simulink model "VehCtrl20260630_18B"  (R2018b)
settings: Solver=FixedStepAuto  StartTime=0.0  StopTime=inf  FixedStep=0.005  RelTol=1e-3
InitFcn:
  | mbd_mpc_consistency_checks(bdroot(gcs));
undefined symbols (not defined in the file): ANG_DEAD, BMS_NormalPwr, BrakeDeadZone, BrkPrsByBrkPct_TB_X, BrkPrsByBrkPct_TB_Y, DELAY_DISCHARGE, DELAY_RCUOFF, DRV_BACKWARD, DRV_BRAKE, DRV_FORWARD, DRV_NEUTRAL, DRV_PARK, DRV_UNPARK, DRV_ZEROTURN, EPB_LOCK, EPB_UNLOCK, ExtraLoadPwr, FanOff, fifo_0_vect, fifo_1_vect, HiFanReq, HV_finished, HV_No_Active, HV_POWER_OFF, HV_POWER_ON, HVDown, HVON, KaTLS_v_DrgUp_X_VehSpd, KeFTM_s_Way1OffDlyTime, KeFTM_TK_Way1CoolLv2OffBatTemp, KeFTM_TK_Way1CoolLv2OffMtrTemp, KeFTM_TK_Way1CoolLv2OnBatTemp, KeFTM_TK_Way1CoolLv2OnMtrTemp, KeFTM_TK_Way1CoolLv3OffBatTemp, KeFTM_TK_Way1CoolLv3OffMtrTemp, KeFTM_TK_Way1CoolLv3OnBatTemp, KeFTM_TK_Way1CoolLv3OnMtrTemp, KeFTM_TK_Way1CoolLv4OffBatTemp, KeFTM_TK_Way1CoolLv4OffMtrTemp, KeFTM_TK_Way1CoolLv4OnBatTemp, KeFTM_TK_Way1CoolLv4OnMtrTemp, Kp1, Kp2, LowFanReq, LQFP, MtrCmdGainFL, MtrCmdGainFR, MtrCmdGainRL, MtrCmdGainRR, MtrPwrFactor_RCU, MtrPwrHighToMidThd, MtrPwrLowToMidThd, MtrPwrMidToHighThd, MtrPwrMidToLowThd, MtrTrqMax, PCT_DEAD, Precharge, PTO_1000, PTO_540, pts1_fifo_0_vect ... (+32)
libraries: mbd_mpc574x_ec_toolbox x175, simulink x110, canmsglib x70
(part 9 of 15)

== system VehCtrl20260630_18B/SigIn/CAN1/BMS_CellVoltageCycTx/UNPACK ==
  ID : Inport
  data : Inport  Port=2
  length : Inport  Port=3
  timestamp : Inport  Port=4
  Action Port : ActionPort  ActionType=case
  Bus Creator : BusCreator  Inputs=7  OutDataTypeStr=Bus: CAN_MESSAGE_BUS  NonVirtualBus=on
  Bus Creator1 : BusCreator  Inputs=5
  CAN Unpack6 : canmsglib/CAN Unpack  CANdbFile=D:\VCU\VCU_AgriculturalMachinery_ChangChun\CAN协议8.4\BMS\BMS_DBC_Sheet1.dbc  MsgList=BMS_CellVoltageCycTx  MsgName=BMS_CellVoltageCycTx  MsgIDType=Extended (29-bit identifier)  MsgIdentifier=404760903  MsgLength=8  SignalInfo=BMS_CellVolGroupNum$12$12$2$2$1$0$1$0$1$4095$#BMS_CellVol_n0$16$12$2$2$1$0$2.000000e-03$0$0$5$#BMS_CellVol_n1$36$12$2$2$1$0$2.000000e-03$0$0$5$#BMS_CellVol_n2$40$12$2$2$1$0$2.000000e-03$0$0$5$#BMS_CellVol_n3$60$12$2$2$1$0$2.000000e-03$0$0$5$#  NSignals=5  IDPort=off  TimestampPort=off  ErrorPort=off  RemotePort=off  LengthPort=off  StatusPort=off  StartBits=str2num('[int32(12);int32(16);int32(36);int32(40);int32(60)]')  SignalSizes=str2num('[int32(12);int32(12);int32(12);int32(12);int32(12)]')  ByteOrders=str2num('[int32(2);int32(2);int32(2);int32(2);int32(2)]')  DataTypes=str2num('[int32(2);int32(2);int32(2);int32(2);int32(2)]')  MultiplexTypes=str2num('[int32(1);int32(1);int32(1);int32(1);int32(1)]')  MultiplexValues=str2num('[double(0);double(0);double(0);double(0);double(0)]')  Factors=str2num('[double(1);double(2.000000e-03);double(2.000000e-03);double(2.000000e-03);double(2.000000e-03)]')  Offsets=str2num('[double(0);double(0);double(0);double(0);double(0)]')  Minimums=str2num('[double(1);double(0);double(0);double(0);double(0)]')  Maximums=str2num('[double(4095);double(5);double(5);double(5);double(5)]')  ApplyMinMax=off
      settings: SourceProductName=Simulink Real-Time  SourceProductBaseCode=XP  DataFormat=CANdb specified signals
  Constant1 : Constant  OutDataTypeStr=uint8
  Constant4 : Constant  Value=0  OutDataTypeStr=uint8
  Constant5 : Constant  Value=0  OutDataTypeStr=uint8
  Data Type Conversion{,14..15,17} (4 alike) : DataTypeConversion  OutDataTypeStr=uint8
  Data Type Conversion{1..4,60} (5 alike) : DataTypeConversion  OutDataTypeStr=single
  Data Type Conversion18 : DataTypeConversion  OutDataTypeStr=uint32
  Data Type Conversion19 : DataTypeConversion  OutDataTypeStr=double
  Message : Outport
  wires:
  Data Type Conversion15/1 -> Bus Creator/3  "Remote"
  Data Type Conversion14/1 -> Bus Creator/2  "Length"
  Data Type Conversion/1 -> Bus Creator/1  "Extended"
  Bus Creator/1 -> CAN Unpack6/1  "CAN_Msg_In"
  Data Type Conversion17/1 -> Bus Creator/4  "Error"
  timestamp/1 -> Data Type Conversion19/1
  Data Type Conversion19/1 -> Bus Creator/6  "Timestamp"
  ID/1 -> Data Type Conversion18/1
  Constant5/1 -> Data Type Conversion17/1
  Constant1/1 -> Data Type Conversion/1
  Data Type Conversion18/1 -> Bus Creator/5  "ID"
  data/1 -> Bus Creator/7  "Data"
  length/1 -> Data Type Conversion14/1
  Constant4/1 -> Data Type Conversion15/1
  CAN Unpack6/1 -> Data Type Conversion1/1
  CAN Unpack6/2 -> Data Type Conversion60/1
  CAN Unpack6/3 -> Data Type Conversion4/1
  CAN Unpack6/4 -> Data Type Conversion3/1
  CAN Unpack6/5 -> Data Type Conversion2/1
  Data Type Conversion1/1 -> Bus Creator1/1  "BMS_CellVolGroupNum"
  Data Type Conversion60/1 -> Bus Creator1/2  "BMS_CellVol_n0"
  Data Type Conversion4/1 -> Bus Creator1/3  "BMS_CellVol_n1"
  Data Type Conversion3/1 -> Bus Creator1/4  "BMS_CellVol_n2"
  Data Type Conversion2/1 -> Bus Creator1/5  "BMS_CellVol_n3"
  Bus Creator1/1 -> Message/1

== system VehCtrl20260630_18B/SigIn/CAN1/BMS_ExtremeCellVoltage/UNPACK ==
  ID : Inport
  data : Inport  Port=2
  length : Inport  Port=3
  timestamp : Inport  Port=4
  Action Port : ActionPort  ActionType=case
  Bus Creator : BusCreator  Inputs=7  OutDataTypeStr=Bus: CAN_MESSAGE_BUS  NonVirtualBus=on
  Bus Creator1 : BusCreator  Inputs=4
  CAN Unpack6 : canmsglib/CAN Unpack  CANdbFile=D:\VCU\VCU_AgriculturalMachinery_ChangChun\CAN协议8.4\BMS\BMS_DBC_Sheet1.dbc  MsgList=BMS_ExtremeCellVoltage  MsgName=BMS_ExtremeCellVoltage  MsgIDType=Extended (29-bit identifier)  MsgIdentifier=402794823  MsgLength=8  SignalInfo=BMS_MaxCellVoltage$16$12$2$2$1$0$2.000000e-03$0$0$5$#BMS_MaxCellVoltageNum$34$10$2$2$1$0$1$0$0$1023$#BMS_MinCellVoltage$54$12$2$2$1$0$2.000000e-03$0$0$5$#BMS_MinCellVoltageNum$56$10$2$2$1$0$1$0$0$1023$#  NSignals=4  IDPort=off  TimestampPort=off  ErrorPort=off  RemotePort=off  LengthPort=off  StatusPort=off  StartBits=str2num('[int32(16);int32(34);int32(54);int32(56)]')  SignalSizes=str2num('[int32(12);int32(10);int32(12);int32(10)]')  ByteOrders=str2num('[int32(2);int32(2);int32(2);int32(2)]')  DataTypes=str2num('[int32(2);int32(2);int32(2);int32(2)]')  MultiplexTypes=str2num('[int32(1);int32(1);int32(1);int32(1)]')  MultiplexValues=str2num('[double(0);double(0);double(0);double(0)]')  Factors=str2num('[double(2.000000e-03);double(1);double(2.000000e-03);double(1)]')  Offsets=str2num('[double(0);double(0);double(0);double(0)]')  Minimums=str2num('[double(0);double(0);double(0);double(0)]')  Maximums=str2num('[double(5);double(1023);double(5);double(1023)]')  ApplyMinMax=off
      settings: SourceProductName=Simulink Real-Time  SourceProductBaseCode=XP  DataFormat=CANdb specified signals
  Constant1 : Constant  OutDataTypeStr=uint8
  Constant4 : Constant  Value=0  OutDataTypeStr=uint8
  Constant5 : Constant  Value=0  OutDataTypeStr=uint8
  Data Type Conversion{,14..15,17} (4 alike) : DataTypeConversion  OutDataTypeStr=uint8
  Data Type Conversion{1..3,60} (4 alike) : DataTypeConversion  OutDataTypeStr=single
  Data Type Conversion18 : DataTypeConversion  OutDataTypeStr=uint32
  Data Type Conversion19 : DataTypeConversion  OutDataTypeStr=double
  Message : Outport
  wires:
  Bus Creator1/1 -> Message/1
  Data Type Conversion15/1 -> Bus Creator/3  "Remote"
  Data Type Conversion14/1 -> Bus Creator/2  "Length"
  Data Type Conversion/1 -> Bus Creator/1  "Extended"
  Bus Creator/1 -> CAN Unpack6/1  "CAN_Msg_In"
  Data Type Conversion17/1 -> Bus Creator/4  "Error"
  timestamp/1 -> Data Type Conversion19/1
  Data Type Conversion19/1 -> Bus Creator/6  "Timestamp"
  ID/1 -> Data Type Conversion18/1
  Constant5/1 -> Data Type Conversion17/1
  Constant1/1 -> Data Type Conversion/1
  Data Type Conversion18/1 -> Bus Creator/5  "ID"
  data/1 -> Bus Creator/7  "Data"
  length/1 -> Data Type Conversion14/1
  Constant4/1 -> Data Type Conversion15/1
  Data Type Conversion3/1 -> Bus Creator1/4  "BMS_MinCellVoltageNum"
  Data Type Conversion2/1 -> Bus Creator1/3  "BMS_MinCellVoltage"
  CAN Unpack6/1 -> Data Type Conversion1/1
  CAN Unpack6/2 -> Data Type Conversion60/1
  CAN Unpack6/4 -> Data Type Conversion3/1
  CAN Unpack6/3 -> Data Type Conversion2/1
  Data Type Conversion1/1 -> Bus Creator1/1  "BMS_MaxCellVoltage"
  Data Type Conversion60/1 -> Bus Creator1/2  "BMS_MaxCellVoltageNum"

== system VehCtrl20260630_18B/SigIn/CAN1/BMS_ExtremeTemp/UNPACK ==
  ID : Inport
  data : Inport  Port=2
  length : Inport  Port=3
  timestamp : Inport  Port=4
  Action Port : ActionPort  ActionType=case
  Bus Creator : BusCreator  Inputs=7  OutDataTypeStr=Bus: CAN_MESSAGE_BUS  NonVirtualBus=on
  Bus Creator1 : BusCreator  Inputs=4
  CAN Unpack6 : canmsglib/CAN Unpack  CANdbFile=D:\VCU\VCU_AgriculturalMachinery_ChangChun\CAN协议8.4\BMS\BMS_DBC_Sheet1.dbc  MsgList=BMS_ExtremeTemp  MsgName=BMS_ExtremeTemp  MsgIDType=Extended (29-bit identifier)  MsgIdentifier=402860359  MsgLength=8  SignalInfo=BMS_MaxBatteryTemp$8$8$2$2$1$0$1$-40$-40$125$#BMS_MaxBatteryTempNum$28$8$2$2$1$0$1$0$0$255$#BMS_MinBatteryTemp$36$8$2$2$1$0$1$-40$-40$125$#BMS_MinBatteryTempNum$40$8$2$2$1$0$1$0$0$255$#  NSignals=4  IDPort=off  TimestampPort=off  ErrorPort=off  RemotePort=off  LengthPort=off  StatusPort=off  StartBits=str2num('[int32(8);int32(28);int32(36);int32(40)]')  SignalSizes=str2num('[int32(8);int32(8);int32(8);int32(8)]')  ByteOrders=str2num('[int32(2);int32(2);int32(2);int32(2)]')  DataTypes=str2num('[int32(2);int32(2);int32(2);int32(2)]')  MultiplexTypes=str2num('[int32(1);int32(1);int32(1);int32(1)]')  MultiplexValues=str2num('[double(0);double(0);double(0);double(0)]')  Factors=str2num('[double(1);double(1);double(1);double(1)]')  Offsets=str2num('[double(-40);double(0);double(-40);double(0)]')  Minimums=str2num('[double(-40);double(0);double(-40);double(0)]')  Maximums=str2num('[double(125);double(255);double(125);double(255)]')  ApplyMinMax=off
      settings: SourceProductName=Simulink Real-Time  SourceProductBaseCode=XP  DataFormat=CANdb specified signals
  Constant1 : Constant  OutDataTypeStr=uint8
  Constant4 : Constant  Value=0  OutDataTypeStr=uint8
  Constant5 : Constant  Value=0  OutDataTypeStr=uint8
  Data Type Conversion{,14..15,17} (4 alike) : DataTypeConversion  OutDataTypeStr=uint8
  Data Type Conversion{1..3,60} (4 alike) : DataTypeConversion  OutDataTypeStr=single
  Data Type Conversion18 : DataTypeConversion  OutDataTypeStr=uint32
  Data Type Conversion19 : DataTypeConversion  OutDataTypeStr=double
  Message : Outport
  wires:
  Bus Creator1/1 -> Message/1
  Data Type Conversion15/1 -> Bus Creator/3  "Remote"
  Data Type Conversion14/1 -> Bus Creator/2  "Length"
  Data Type Conversion/1 -> Bus Creator/1  "Extended"
  Bus Creator/1 -> CAN Unpack6/1  "CAN_Msg_In"
  Data Type Conversion17/1 -> Bus Creator/4  "Error"
  timestamp/1 -> Data Type Conversion19/1
  Data Type Conversion19/1 -> Bus Creator/6  "Timestamp"
  ID/1 -> Data Type Conversion18/1
  Constant5/1 -> Data Type Conversion17/1
  Constant1/1 -> Data Type Conversion/1
  Data Type Conversion18/1 -> Bus Creator/5  "ID"
  data/1 -> Bus Creator/7  "Data"
  length/1 -> Data Type Conversion14/1
  Constant4/1 -> Data Type Conversion15/1
  CAN Unpack6/4 -> Data Type Conversion3/1
  CAN Unpack6/3 -> Data Type Conversion2/1
  CAN Unpack6/2 -> Data Type Conversion1/1
  CAN Unpack6/1 -> Data Type Conversion60/1
  Data Type Conversion60/1 -> Bus Creator1/1  "BMS_MaxBatteryTemp"
  Data Type Conversion1/1 -> Bus Creator1/2  "BMS_MaxBatteryTempNum"
  Data Type Conversion2/1 -> Bus Creator1/3  "BMS_MinBatteryTemp"
  Data Type Conversion3/1 -> Bus Creator1/4  "BMS_MinBatteryTempNum"

== system VehCtrl20260630_18B/SigIn/CAN1/BMS_PackCalc/UNPACK ==
  ID : Inport
  data : Inport  Port=2
  length : Inport  Port=3
  timestamp : Inport  Port=4
  Action Port : ActionPort  ActionType=case
  Add : Sum
  Bus Creator : BusCreator  Inputs=7  OutDataTypeStr=Bus: CAN_MESSAGE_BUS  NonVirtualBus=on
  Bus Creator1 : BusCreator  Inputs=3
  CAN Unpack6 : canmsglib/CAN Unpack  CANdbFile=D:\VCU\VCU_AgriculturalMachinery_ChangChun\CAN协议8.4\BMS\BMS_DBC_Sheet1.dbc  MsgList=BMS_PackCalc  MsgName=BMS_PackCalc  MsgIDType=Extended (29-bit identifier)  MsgIdentifier=402991431  MsgLength=8  SignalInfo=BMS_NegInsulation$56$16$2$2$1$0$1$0$0$60000$#BMS_PosInsulation$40$16$2$2$1$0$1$0$0$60000$#BMS_SupplyVol$24$8$2$2$1$0$5.000000e-01$0$0$36$#  NSignals=3  IDPort=off  TimestampPort=off  ErrorPort=off  RemotePort=off  LengthPort=off  StatusPort=off  StartBits=str2num('[int32(56);int32(40);int32(24)]')  SignalSizes=str2num('[int32(16);int32(16);int32(8)]')  ByteOrders=str2num('[int32(2);int32(2);int32(2)]')  DataTypes=str2num('[int32(2);int32(2);int32(2)]')  MultiplexTypes=str2num('[int32(1);int32(1);int32(1)]')  MultiplexValues=str2num('[double(0);double(0);double(0)]')  Factors=str2num('[double(1);double(1);double(5.000000e-01)]')  Offsets=str2num('[double(0);double(0);double(0)]')  Minimums=str2num('[double(0);double(0);double(0)]')  Maximums=str2num('[double(60000);double(60000);double(36)]')  ApplyMinMax=off
      settings: SourceProductName=Simulink Real-Time  SourceProductBaseCode=XP  DataFormat=CANdb specified signals
  Constant : Constant  OutDataTypeStr=uint8
  Constant1 : Constant  OutDataTypeStr=uint8
  Constant4 : Constant  Value=0  OutDataTypeStr=uint8
  Constant5 : Constant  Value=0  OutDataTypeStr=uint8
  Data Store Read : DataStoreRead  DataStoreName=Cnt_BMS3
  Data Store Write : DataStoreWrite  DataStoreName=Cnt_BMS3
  Data Type Conversion{,14..15,17} (4 alike) : DataTypeConversion  OutDataTypeStr=uint8
  Data Type Conversion18 : DataTypeConversion  OutDataTypeStr=uint32
  Data Type Conversion19 : DataTypeConversion  OutDataTypeStr=double
  Data Type Conversion41 : DataTypeConversion  OutDataTypeStr=single
  Data Type Conversion44 : DataTypeConversion  OutDataTypeStr=single
  Data Type Conversion45 : DataTypeConversion  OutDataTypeStr=single
  Message : Outport
  wires:
  Data Type Conversion44/1 -> Bus Creator1/2  "BMS_PosInsulation"
  Data Type Conversion41/1 -> Bus Creator1/1  "BMS_SupplyVol"
  Bus Creator1/1 -> Message/1
  Data Type Conversion15/1 -> Bus Creator/3  "Remote"
  Data Type Conversion14/1 -> Bus Creator/2  "Length"
  Data Type Conversion/1 -> Bus Creator/1  "Extended"
  Bus Creator/1 -> CAN Unpack6/1  "CAN_Msg_In"
  Data Type Conversion17/1 -> Bus Creator/4  "Error"
  timestamp/1 -> Data Type Conversion19/1
  Data Type Conversion19/1 -> Bus Creator/6  "Timestamp"
  ID/1 -> Data Type Conversion18/1
  Constant5/1 -> Data Type Conversion17/1
  Constant1/1 -> Data Type Conversion/1
  Data Type Conversion18/1 -> Bus Creator/5  "ID"
  data/1 -> Bus Creator/7  "Data"
  length/1 -> Data Type Conversion14/1
  Constant4/1 -> Data Type Conversion15/1
  Data Type Conversion45/1 -> Bus Creator1/3  "BMS_NegInsulation"
  CAN Unpack6/1 -> Data Type Conversion45/1
  CAN Unpack6/2 -> Data Type Conversion44/1
  CAN Unpack6/3 -> Data Type Conversion41/1
  Add/1 -> Data Store Write/1
  Constant/1 -> Add/2
  Data Store Read/1 -> Add/1

== system VehCtrl20260630_18B/SigIn/CAN1/BMS_PackLimitPower/UNPACK ==
  ID : Inport
  data : Inport  Port=2
  length : Inport  Port=3
  timestamp : Inport  Port=4
  Action Port : ActionPort  ActionType=case
  Add : Sum
  Bus Creator : BusCreator  Inputs=7  OutDataTypeStr=Bus: CAN_MESSAGE_BUS  NonVirtualBus=on
  Bus Creator1 : BusCreator  Inputs=4
  CAN Unpack6 : canmsglib/CAN Unpack  CANdbFile=D:\VCU\VCU_AgriculturalMachinery_ChangChun\CAN协议8.4\BMS\BMS_DBC_Sheet1.dbc  MsgList=BMS_PackLimitPower  MsgName=BMS_PackLimitPower  MsgIDType=Extended (29-bit identifier)  MsgIdentifier=403056967  MsgLength=8  SignalInfo=BMS_MaxLimitDisChargeCurrent$40$16$2$2$1$0$1.000000e-01$-2000$-2000$2000$#BMS_MaxLimitDisChargePower$8$16$2$2$1$0$1.000000e-01$0$0$3000$#BMS_MaxLimitReChargeCurrent$56$16$2$2$1$0$1.000000e-01$-2000$-2000$-2000$#BMS_MaxLimitReChargePower$24$16$2$2$1$0$1.000000e-01$0$0$3000$#  NSignals=4  IDPort=off  TimestampPort=off  ErrorPort=off  RemotePort=off  LengthPort=off  StatusPort=off  StartBits=str2num('[int32(40);int32(8);int32(56);int32(24)]')  SignalSizes=str2num('[int32(16);int32(16);int32(16);int32(16)]')  ByteOrders=str2num('[int32(2);int32(2);int32(2);int32(2)]')  DataTypes=str2num('[int32(2);int32(2);int32(2);int32(2)]')  MultiplexTypes=str2num('[int32(1);int32(1);int32(1);int32(1)]')  MultiplexValues=str2num('[double(0);double(0);double(0);double(0)]')  Factors=str2num('[double(1.000000e-01);double(1.000000e-01);double(1.000000e-01);double(1.000000e-01)]')  Offsets=str2num('[double(-2000);double(0);double(-2000);double(0)]')  Minimums=str2num('[double(-2000);double(0);double(-2000);double(0)]')  Maximums=str2num('[double(2000);double(3000);double(-2000);double(3000)]')  ApplyMinMax=off
      settings: SourceProductName=Simulink Real-Time  SourceProductBaseCode=XP  DataFormat=CANdb specified signals
  Constant : Constant  OutDataTypeStr=uint8
  Constant1 : Constant  OutDataTypeStr=uint8
  Constant4 : Constant  Value=0  OutDataTypeStr=uint8
  Constant5 : Constant  Value=0  OutDataTypeStr=uint8
  Data Store Read : DataStoreRead  DataStoreName=Cnt_BMS4
  Data Store Write : DataStoreWrite  DataStoreName=Cnt_BMS4
  Data Type Conversion{,14..15,17} (4 alike) : DataTypeConversion  OutDataTypeStr=uint8
  Data Type Conversion18 : DataTypeConversion  OutDataTypeStr=uint32
  Data Type Conversion19 : DataTypeConversion  OutDataTypeStr=double
  Data Type Conversion{60..63} (4 alike) : DataTypeConversion  OutDataTypeStr=single
  Message : Outport
  wires:
  Constant4/1 -> Data Type Conversion15/1
  length/1 -> Data Type Conversion14/1
  data/1 -> Bus Creator/7  "Data"
  Data Type Conversion18/1 -> Bus Creator/5  "ID"
  Constant1/1 -> Data Type Conversion/1
  Constant5/1 -> Data Type Conversion17/1
  ID/1 -> Data Type Conversion18/1
  Data Type Conversion19/1 -> Bus Creator/6  "Timestamp"
  timestamp/1 -> Data Type Conversion19/1
  Data Type Conversion17/1 -> Bus Creator/4  "Error"
  Bus Creator/1 -> CAN Unpack6/1  "CAN_Msg_In"
  Data Type Conversion/1 -> Bus Creator/1  "Extended"
  Data Type Conversion14/1 -> Bus Creator/2  "Length"
  Data Type Conversion15/1 -> Bus Creator/3  "Remote"
  Bus Creator1/1 -> Message/1
  Data Type Conversion60/1 -> Bus Creator1/1  "BMS_MaxLimitDisChargePower"
  Data Type Conversion61/1 -> Bus Creator1/2  "BMS_MaxLimitReChargePower"
  Data Type Conversion62/1 -> Bus Creator1/3  "BMS_MaxLimitDisChargeCurrent"
  Data Type Conversion63/1 -> Bus Creator1/4  "BMS_MaxLimitReChargeCurrent"
  CAN Unpack6/2 -> Data Type Conversion60/1
  CAN Unpack6/1 -> Data Type Conversion62/1
  CAN Unpack6/3 -> Data Type Conversion63/1
  CAN Unpack6/4 -> Data Type Conversion61/1
  Add/1 -> Data Store Write/1
  Constant/1 -> Add/2
  Data Store Read/1 -> Add/1

== system VehCtrl20260630_18B/SigIn/CAN1/BMS_PackMeasure/UNPACK ==
  ID : Inport
  data : Inport  Port=2
  length : Inport  Port=3
  timestamp : Inport  Port=4
  Action Port : ActionPort  ActionType=case
  Add : Sum
  Bus Creator : BusCreator  Inputs=7  OutDataTypeStr=Bus: CAN_MESSAGE_BUS  NonVirtualBus=on
  Bus Creator1 : BusCreator  Inputs=2
  CAN Unpack6 : canmsglib/CAN Unpack  CANdbFile=D:\VCU\VCU_AgriculturalMachinery_ChangChun\CAN协议8.4\BMS\BMS_DBC_Sheet1.dbc  MsgList=BMS_PackMeasure  MsgName=BMS_PackMeasure  MsgIDType=Extended (29-bit identifier)  MsgIdentifier=402729287  MsgLength=8  SignalInfo=BMS_LineVoltage$40$16$2$2$1$0$1.000000e-01$0$0$2000$#BMS_PackCurrent$8$16$2$2$1$0$1.000000e-01$-2000$-2000$2000$#  NSignals=2  IDPort=off  TimestampPort=off  ErrorPort=off  RemotePort=off  LengthPort=off  StatusPort=off  StartBits=str2num('[int32(40);int32(8)]')  SignalSizes=str2num('[int32(16);int32(16)]')  ByteOrders=str2num('[int32(2);int32(2)]')  DataTypes=str2num('[int32(2);int32(2)]')  MultiplexTypes=str2num('[int32(1);int32(1)]')  MultiplexValues=str2num('[double(0);double(0)]')  Factors=str2num('[double(1.000000e-01);double(1.000000e-01)]')  Offsets=str2num('[double(0);double(-2000)]')  Minimums=str2num('[double(0);double(-2000)]')  Maximums=str2num('[double(2000);double(2000)]')  ApplyMinMax=off
      settings: SourceProductName=Simulink Real-Time  SourceProductBaseCode=XP  DataFormat=CANdb specified signals
  Constant : Constant  OutDataTypeStr=uint8
  Constant1 : Constant  OutDataTypeStr=uint8
  Constant4 : Constant  Value=0  OutDataTypeStr=uint8
  Constant5 : Constant  Value=0  OutDataTypeStr=uint8
  Data Store Read : DataStoreRead  DataStoreName=Cnt_BMS1
  Data Store Write : DataStoreWrite  DataStoreName=Cnt_BMS1
  Data Type Conversion{,14..15,17} (4 alike) : DataTypeConversion  OutDataTypeStr=uint8
  Data Type Conversion18 : DataTypeConversion  OutDataTypeStr=uint32
  Data Type Conversion19 : DataTypeConversion  OutDataTypeStr=double
  Data Type Conversion60 : DataTypeConversion  OutDataTypeStr=single
  Data Type Conversion61 : DataTypeConversion  OutDataTypeStr=single
  Message : Outport
  wires:
  Data Type Conversion61/1 -> Bus Creator1/1  "BMS_LineVoltage"
  Data Type Conversion60/1 -> Bus Creator1/2  "BMS_PackCurrent"
  Bus Creator1/1 -> Message/1
  Data Type Conversion15/1 -> Bus Creator/3  "Remote"
  Data Type Conversion14/1 -> Bus Creator/2  "Length"
  Data Type Conversion/1 -> Bus Creator/1  "Extended"
  Bus Creator/1 -> CAN Unpack6/1  "CAN_Msg_In"
  Data Type Conversion17/1 -> Bus Creator/4  "Error"
  timestamp/1 -> Data Type Conversion19/1
  Data Type Conversion19/1 -> Bus Creator/6  "Timestamp"
  ID/1 -> Data Type Conversion18/1
  Constant5/1 -> Data Type Conversion17/1
  Constant1/1 -> Data Type Conversion/1
  Data Type Conversion18/1 -> Bus Creator/5  "ID"
  data/1 -> Bus Creator/7  "Data"
  length/1 -> Data Type Conversion14/1
  Constant4/1 -> Data Type Conversion15/1
  CAN Unpack6/1 -> Data Type Conversion61/1
  CAN Unpack6/2 -> Data Type Conversion60/1
  Data Store Read/1 -> Add/1
  Add/1 -> Data Store Write/1
  Constant/1 -> Add/2

== system VehCtrl20260630_18B/SigIn/CAN1/BMS_PackStateInf/UNPACK ==
  ID : Inport
  data : Inport  Port=2
  length : Inport  Port=3
  timestamp : Inport  Port=4
  Action Port : ActionPort  ActionType=case
  Add : Sum
  Bus Creator : BusCreator  Inputs=7  OutDataTypeStr=Bus: CAN_MESSAGE_BUS  NonVirtualBus=on
  Bus Creator1 : BusCreator  Inputs=5
  CAN Unpack6 : canmsglib/CAN Unpack  CANdbFile=D:\VCU\VCU_AgriculturalMachinery_ChangChun\CAN协议8.4\BMS\BMS_DBC_Sheet1.dbc  MsgList=BMS_PackStateInf  MsgName=BMS_PackStateInf  MsgIDType=Extended (29-bit identifier)  MsgIdentifier=402925895  MsgLength=8  SignalInfo=BMS_BatteryChargeState$4$4$2$2$1$0$1$0$0$5$#BMS_BatteryState$0$4$2$2$1$0$1$0$0$5$#BMS_CellVoltageDiffFaultFlag$50$1$2$2$1$0$1$0$0$1$#BMS_CellVoltageHighFaultFlag$45$1$2$2$1$0$1$0$0$1$#BMS_CellVoltageLowFaultFlag$46$1$2$2$1$0$1$0$0$1$#BMS_ChrgVoltageHighFaultFlag$53$1$2$2$1$0$1$0$0$1$#BMS_FaultCode$32$16$2$2$1$0$1$0$0$65535$#BMS_FaultLevel$16$4$2$2$1$0$1$0$0$15$#BMS_FaultNum$20$4$2$2$1$0$1$0$0$15$#BMS_FullChargSts$54$1$2$2$1$0$1$0$0$1$#BMS_HVLockFaultFlag$52$1$2$2$1$0$1$0$0$1$#BMS_MaxChginterfaceTemp$8$8$2$2$1$0$1$-40$-40$125$#BMS_PackVoltageHighFaultFlag$42$1$2$2$1$0$1$0$0$1$#BMS_PackVoltageLowFaultFlag$43$1$2$2$1$0$1$0$0$1$#BMS_SOCHighFaultFlag$47$1$2$2$1$0$1$0$0$1$#BMS_SOCJumpFaultFlag$48$1$2$2$1$0$1$0$0$1$#BMS_SOCLowFaultFlag$44$1$2$2$1$0$1$0$0$1$#BMS_SysInsulationFaultFlag$51$1$2$2$1$0$1$0$0$1$#BMS_SysNoMatchFaultFlag$49$1$2$2$1$0$1$0$0$1$#BMS_TempDiffFaultFlag$40$1$2$2$1$0$1$0$0$1$#BMS_TempHighFaultFlag$41$1$2$2$1$0$1$0$0$1$#  NSignals=21  IDPort=off  TimestampPort=off  ErrorPort=off  RemotePort=off  LengthPort=off  StatusPort=off  StartBits=str2num('[int32(4);int32(0);int32(50);int32(45);int32(46);int32(53);int32(32);int32(16);int32(20);int32(54);int32(52);int32(8);int32(42);int32(43);int32(47);int32(48);int32(44);int32(51);int32(49);int32(40);int32(41)]')  SignalSizes=str2num('[int32(4);int32(4);int32(1);int32(1);int32(1);int32(1);int32(16);int32(4);int32(4);int32(1);int32(1);int32(8);int32(1);int32(1);int32(1);int32(1);int32(1);int32(1);int32(1);int32(1);int32(1)]')  ByteOrders=str2num('[int32(2);int32(2);int32(2);int32(2);int32(2);int32(2);int32(2);int32(2);int32(2);int32(2);int32(2);int32(2);int32(2);int32(2);int32(2);int32(2);int32(2);int32(2);int32(2);int32(2);int32(2)]')  DataTypes=str2num('[int32(2);int32(2);int32(2);int32(2);int32(2);int32(2);int32(2);int32(2);int32(2);int32(2);int32(2);int32(2);int32(2);int32(2);int32(2);int32(2);int32(2);int32(2);int32(2);int32(2);int32(2)]')  MultiplexTypes=str2num('[int32(1);int32(1);int32(1);int32(1);int32(1);int32(1);int32(1);int32(1);int32(1);int32(1);int32(1);int32(1);int32(1);int32(1);int32(1);int32(1);int32(1);int32(1);int32(1);int32(1);int32(1)]')  MultiplexValues=str2num('[double(0);double(0);double(0);double(0);double(0);double(0);double(0);double(0);double(0);double(0);double(0);double(0);double(0);double(0);double(0);double(0);double(0);double(0);double(0);double(0);double(0)]')  Factors=str2num('[double(1);double(1);double(1);double(1);double(1);double(1);double(1);double(1);double(1);double(1);double(1);double(1);double(1);double(1);double(1);double(1);double(1);double(1);double(1);double(1);double(1)]')  Offsets=str2num('[double(0);double(0);double(0);double(0);double(0);double(0);double(0);double(0);double(0);double(0);double(0);double(-40);double(0);double(0);double(0);double(0);double(0);double(0);double(0);double(0);double(0)]')  Minimums=str2num('[double(0);double(0);double(0);double(0);double(0);double(0);double(0);double(0);double(0);double(0);double(0);double(-40);double(0);double(0);double(0);double(0);double(0);double(0);double(0);double(0);double(0)]')  Maximums=str2num('[double(5);double(5);double(1);double(1);double(1);double(1);double(65535);double(15);double(15);double(1);double(1);double(125);double(1);double(1);double(1);double(1);double(1);double(1);double(1);double(1);double(1)]')  ApplyMinMax=off
      settings: SourceProductName=Simulink Real-Time  SourceProductBaseCode=XP  DataFormat=CANdb specified signals
  Constant : Constant  OutDataTypeStr=uint8
  Constant1 : Constant  OutDataTypeStr=uint8
  Constant4 : Constant  Value=0  OutDataTypeStr=uint8
  Constant5 : Constant  Value=0  OutDataTypeStr=uint8
  Data Store Read : DataStoreRead  DataStoreName=Cnt_BMS2
  Data Store Write : DataStoreWrite  DataStoreName=Cnt_BMS2
  Data Type Conversion{,1..2,14..15,17,60,63} (8 alike) : DataTypeConversion  OutDataTypeStr=uint8
  Data Type Conversion18 : DataTypeConversion  OutDataTypeStr=uint32
  Data Type Conversion19 : DataTypeConversion  OutDataTypeStr=double
  Data Type Conversion62 : DataTypeConversion  OutDataTypeStr=single
  Terminator{,1..15} (16 alike) : Terminator
  Message : Outport
  wires:
  Constant4/1 -> Data Type Conversion15/1
  length/1 -> Data Type Conversion14/1
  data/1 -> Bus Creator/7  "Data"
  Data Type Conversion18/1 -> Bus Creator/5  "ID"
  Constant1/1 -> Data Type Conversion/1
  Constant5/1 -> Data Type Conversion17/1
  ID/1 -> Data Type Conversion18/1
  Data Type Conversion19/1 -> Bus Creator/6  "Timestamp"
  timestamp/1 -> Data Type Conversion19/1
  Data Type Conversion17/1 -> Bus Creator/4  "Error"
  Bus Creator/1 -> CAN Unpack6/1  "CAN_Msg_In"
  Data Type Conversion/1 -> Bus Creator/1  "Extended"
  Data Type Conversion14/1 -> Bus Creator/2  "Length"
  Data Type Conversion15/1 -> Bus Creator/3  "Remote"
  Bus Creator1/1 -> Message/1
  Data Type Conversion60/1 -> Bus Creator1/1  "BMS_BatteryState"
  Data Type Conversion2/1 -> Bus Creator1/2  "BMS_BatteryChargeState"
  Data Type Conversion62/1 -> Bus Creator1/3  "BMS_MaxChginterfaceTemp"
  Data Type Conversion63/1 -> Bus Creator1/4  "BMS_FaultLevel"
  Data Type Conversion1/1 -> Bus Creator1/5  "BMS_FullChargSts"
  CAN Unpack6/2 -> Data Type Conversion60/1
  CAN Unpack6/1 -> Data Type Conversion2/1
  CAN Unpack6/12 -> Data Type Conversion62/1
  CAN Unpack6/8 -> Data Type Conversion63/1
  CAN Unpack6/10 -> Data Type Conversion1/1
  CAN Unpack6/21 -> Terminator/1
  CAN Unpack6/20 -> Terminator1/1
  CAN Unpack6/19 -> Terminator2/1
  CAN Unpack6/18 -> Terminator3/1
  CAN Unpack6/17 -> Terminator4/1
  CAN Unpack6/16 -> Terminator5/1
  CAN Unpack6/15 -> Terminator6/1
  CAN Unpack6/14 -> Terminator7/1
  CAN Unpack6/13 -> Terminator8/1
  CAN Unpack6/11 -> Terminator9/1
  CAN Unpack6/9 -> Terminator10/1
  CAN Unpack6/7 -> Terminator11/1
  CAN Unpack6/6 -> Terminator12/1  "MCU_RollingCounter"
  CAN Unpack6/5 -> Terminator13/1
  CAN Unpack6/4 -> Terminator14/1
  CAN Unpack6/3 -> Terminator15/1
  Add/1 -> Data Store Write/1
  Constant/1 -> Add/2
  Data Store Read/1 -> Add/1

== system VehCtrl20260630_18B/SigIn/CAN1/BMS_Relaystatus/UNPACK ==
  ID : Inport
  data : Inport  Port=2
  length : Inport  Port=3
  timestamp : Inport  Port=4
  Action Port : ActionPort  ActionType=case
  Bus Creator : BusCreator  Inputs=7  OutDataTypeStr=Bus: CAN_MESSAGE_BUS  NonVirtualBus=on
  Bus Creator1 : BusCreator  Inputs=2
  CAN Unpack6 : canmsglib/CAN Unpack  CANdbFile=D:\VCU\VCU_AgriculturalMachinery_ChangChun\CAN协议8.4\BMS\BMS_DBC_Sheet1.dbc  MsgList=BMS_Relaystatus  MsgName=BMS_Relaystatus  MsgIDType=Extended (29-bit identifier)  MsgIdentifier=471823687  MsgLength=8  SignalInfo=ESM_attachment1justRelay$15$1$2$2$1$0$1$0$0$1$#ESM_chargingnegative1relay$0$1$2$2$1$0$1$0$0$1$#  NSignals=2  IDPort=off  TimestampPort=off  ErrorPort=off  RemotePort=off  LengthPort=off  StatusPort=off  StartBits=str2num('[int32(15);int32(0)]')  SignalSizes=str2num('[int32(1);int32(1)]')  ByteOrders=str2num('[int32(2);int32(2)]')  DataTypes=str2num('[int32(2);int32(2)]')  MultiplexTypes=str2num('[int32(1);int32(1)]')  MultiplexValues=str2num('[double(0);double(0)]')  Factors=str2num('[double(1);double(1)]')  Offsets=str2num('[double(0);double(0)]')  Minimums=str2num('[double(0);double(0)]')  Maximums=str2num('[double(1);double(1)]')  ApplyMinMax=off
      settings: SourceProductName=Simulink Real-Time  SourceProductBaseCode=XP  DataFormat=CANdb specified signals
  Constant1 : Constant  OutDataTypeStr=uint8
  Constant4 : Constant  Value=0  OutDataTypeStr=uint8
  Constant5 : Constant  Value=0  OutDataTypeStr=uint8
  Data Type Conversion{,1,14..15,17,60} (6 alike) : DataTypeConversion  OutDataTypeStr=uint8
  Data Type Conversion18 : DataTypeConversion  OutDataTypeStr=uint32
  Data Type Conversion19 : DataTypeConversion  OutDataTypeStr=double
  Message : Outport
  wires:
  Bus Creator1/1 -> Message/1
  Data Type Conversion15/1 -> Bus Creator/3  "Remote"
  Data Type Conversion14/1 -> Bus Creator/2  "Length"
  Data Type Conversion/1 -> Bus Creator/1  "Extended"
  Bus Creator/1 -> CAN Unpack6/1  "CAN_Msg_In"
  Data Type Conversion17/1 -> Bus Creator/4  "Error"
  timestamp/1 -> Data Type Conversion19/1
  Data Type Conversion19/1 -> Bus Creator/6  "Timestamp"
  ID/1 -> Data Type Conversion18/1
  Constant5/1 -> Data Type Conversion17/1
  Constant1/1 -> Data Type Conversion/1
  Data Type Conversion18/1 -> Bus Creator/5  "ID"
  data/1 -> Bus Creator/7  "Data"
  length/1 -> Data Type Conversion14/1
  Constant4/1 -> Data Type Conversion15/1
  Data Type Conversion1/1 -> Bus Creator1/2  "ESM_attachment1justRelay"
  Data Type Conversion60/1 -> Bus Creator1/1  "ESM_chargingnegative1relay"
  CAN Unpack6/2 -> Data Type Conversion1/1
  CAN Unpack6/1 -> Data Type Conversion60/1

== system VehCtrl20260630_18B/SigIn/CAN1/DbugBMS_ESM/UNPACK ==
  ID : Inport
  data : Inport  Port=2
  length : Inport  Port=3
  timestamp : Inport  Port=4
  Action Port : ActionPort  ActionType=case
  Bus Creator : BusCreator  Inputs=7  OutDataTypeStr=Bus: CAN_MESSAGE_BUS  NonVirtualBus=on
  Bus Creator1 : BusCreator  Inputs=17
  CAN Unpack6 : canmsglib/CAN Unpack  CANdbFile=D:\VCU\VCU_AgriculturalMachinery_ChangChun\CAN协议8.4\BMS\BMS_DBC_Sheet1.dbc  MsgList=DbugBMS_ESM  MsgName=DbugBMS_ESM  MsgIDType=Extended (29-bit identifier)  MsgIdentifier=470185287  MsgLength=8  SignalInfo=EDM_ErrLevPDownNow$1$1$2$2$1$0$1$0$0$1$#EDM_ErrPDownDelay$0$1$2$2$1$0$1$0$0$1$#EDM_NoChrg$4$1$2$2$1$0$1$0$0$1$#EDM_NoHeating$3$1$2$2$1$0$1$0$0$1$#EDM_NoPUp$2$1$2$2$1$0$1$0$0$1$#ESM_BMSChargSts$56$4$2$2$1$0$1$0$0$15$#ESM_BMSWrkSts$60$4$2$2$1$0$1$0$0$15$#ESM_DCChgRelaySt$52$1$2$2$1$0$1$0$0$1$#ESM_FullChargSts$55$1$2$2$1$0$1$0$0$1$#ESM_NegRelaySt$49$1$2$2$1$0$1$0$0$1$#ESM_PUDSt$8$8$2$2$1$0$1$0$0$1$#ESM_PUDTimer$40$32$2$2$1$0$1$0$0$4294967295$#ESM_PosRelaySt$48$1$2$2$1$0$1$0$0$1$#ESM_PreRelaySt$50$1$2$2$1$0$1$0$0$1$#IPI_CC2St$7$1$2$2$1$0$1$0$0$1$#IPI_ChrgSignal$6$1$2$2$1$0$1$0$0$1$#IPI_KeySignal$5$1$2$2$1$0$1$0$0$1$#  NSignals=17  IDPort=off  TimestampPort=off  ErrorPort=off  RemotePort=off  LengthPort=off  StatusPort=off  StartBits=str2num('[int32(1);int32(0);int32(4);int32(3);int32(2);int32(56);int32(60);int32(52);int32(55);int32(49);int32(8);int32(40);int32(48);int32(50);int32(7);int32(6);int32(5)]')  SignalSizes=str2num('[int32(1);int32(1);int32(1);int32(1);int32(1);int32(4);int32(4);int32(1);int32(1);int32(1);int32(8);int32(32);int32(1);int32(1);int32(1);int32(1);int32(1)]')  ByteOrders=str2num('[int32(2);int32(2);int32(2);int32(2);int32(2);int32(2);int32(2);int32(2);int32(2);int32(2);int32(2);int32(2);int32(2);int32(2);int32(2);int32(2);int32(2)]')  DataTypes=str2num('[int32(2);int32(2);int32(2);int32(2);int32(2);int32(2);int32(2);int32(2);int32(2);int32(2);int32(2);int32(2);int32(2);int32(2);int32(2);int32(2);int32(2)]')  MultiplexTypes=str2num('[int32(1);int32(1);int32(1);int32(1);int32(1);int32(1);int32(1);int32(1);int32(1);int32(1);int32(1);int32(1);int32(1);int32(1);int32(1);int32(1);int32(1)]')  MultiplexValues=str2num('[double(0);double(0);double(0);double(0);double(0);double(0);double(0);double(0);double(0);double(0);double(0);double(0);double(0);double(0);double(0);double(0);double(0)]')  Factors=str2num('[double(1);double(1);double(1);double(1);double(1);double(1);double(1);double(1);double(1);double(1);double(1);double(1);double(1);double(1);double(1);double(1);double(1)]')  Offsets=str2num('[double(0);double(0);double(0);double(0);double(0);double(0);double(0);double(0);double(0);double(0);double(0);double(0);double(0);double(0);double(0);double(0);double(0)]')  Minimums=str2num('[double(0);double(0);double(0);double(0);double(0);double(0);double(0);double(0);double(0);double(0);double(0);double(0);double(0);double(0);double(0);double(0);double(0)]')  Maximums=str2num('[double(1);double(1);double(1);double(1);double(1);double(15);double(15);double(1);double(1);double(1);double(1);double(4294967295);double(1);double(1);double(1);double(1);double(1)]')  ApplyMinMax=off
      settings: SourceProductName=Simulink Real-Time  SourceProductBaseCode=XP  DataFormat=CANdb specified signals
  Constant1 : Constant  OutDataTypeStr=uint8
  Constant4 : Constant  Value=0  OutDataTypeStr=uint8
  Constant5 : Constant  Value=0  OutDataTypeStr=uint8
  Data Type Conversion{,1..17,20,23,60} (21 alike) : DataTypeConversion  OutDataTypeStr=uint8
  Data Type Conversion18 : DataTypeConversion  OutDataTypeStr=uint32
  Data Type Conversion19 : DataTypeConversion  OutDataTypeStr=double
  Message : Outport
  wires:
  Bus Creator1/1 -> Message/1
  Data Type Conversion15/1 -> Bus Creator/3  "Remote"
  Data Type Conversion14/1 -> Bus Creator/2  "Length"
  Data Type Conversion/1 -> Bus Creator/1  "Extended"
  Bus Creator/1 -> CAN Unpack6/1  "CAN_Msg_In"
  Data Type Conversion17/1 -> Bus Creator/4  "Error"
  timestamp/1 -> Data Type Conversion19/1
  Data Type Conversion19/1 -> Bus Creator/6  "Timestamp"
  ID/1 -> Data Type Conversion18/1
  Constant5/1 -> Data Type Conversion17/1
  Constant1/1 -> Data Type Conversion/1
  Data Type Conversion18/1 -> Bus Creator/5  "ID"
  data/1 -> Bus Creator/7  "Data"
  length/1 -> Data Type Conversion14/1
  Constant4/1 -> Data Type Conversion15/1
  Data Type Conversion20/1 -> Bus Creator1/14  "ESM_DCChgRelaySt"
  Data Type Conversion13/1 -> Bus Creator1/15  "ESM_FullChargSts"
  Data Type Conversion7/1 -> Bus Creator1/9  "ESM_PUDSt"
  Data Type Conversion10/1 -> Bus Creator1/12  "ESM_NegRelaySt"
  Data Type Conversion8/1 -> Bus Creator1/11  "ESM_PosRelaySt"
  Data Type Conversion5/1 -> Bus Creator1/7  "IPI_ChrgSignal"
  Data Type Conversion6/1 -> Bus Creator1/8  "IPI_CC2St"
  Data Type Conversion3/1 -> Bus Creator1/4  "EDM_NoHeating"
  Data Type Conversion2/1 -> Bus Creator1/3  "EDM_NoPUp"
  Data Type Conversion4/1 -> Bus Creator1/5  "EDM_NoChrg"
  Data Type Conversion11/1 -> Bus Creator1/10  "ESM_PUDTimer"
  Data Type Conversion23/1 -> Bus Creator1/16  "ESM_BMSChargSts"
  Data Type Conversion1/1 -> Bus Creator1/2  "EDM_ErrLevPDownNow"
  Data Type Conversion16/1 -> Bus Creator1/13  "ESM_PreRelaySt"
  Data Type Conversion9/1 -> Bus Creator1/6  "IPI_KeySignal"
  Data Type Conversion12/1 -> Bus Creator1/17  "ESM_BMSWrkSts"
  Data Type Conversion60/1 -> Bus Creator1/1  "EDM_ErrPDownDelay"
  CAN Unpack6/1 -> Data Type Conversion1/1  "MCU_FaultLevel"
  CAN Unpack6/2 -> Data Type Conversion60/1  "MCU_FaultNumber"
  CAN Unpack6/3 -> Data Type Conversion4/1
  CAN Unpack6/4 -> Data Type Conversion3/1
  CAN Unpack6/5 -> Data Type Conversion2/1
  CAN Unpack6/6 -> Data Type Conversion23/1  "MCU_RollingCounter"
  CAN Unpack6/7 -> Data Type Conversion12/1
  CAN Unpack6/8 -> Data Type Conversion20/1
  CAN Unpack6/9 -> Data Type Conversion13/1
  CAN Unpack6/10 -> Data Type Conversion10/1
  CAN Unpack6/11 -> Data Type Conversion7/1
  CAN Unpack6/12 -> Data Type Conversion11/1
  CAN Unpack6/13 -> Data Type Conversion8/1
  CAN Unpack6/14 -> Data Type Conversion16/1
  CAN Unpack6/15 -> Data Type Conversion6/1
  CAN Unpack6/16 -> Data Type Conversion5/1
  CAN Unpack6/17 -> Data Type Conversion9/1

== system VehCtrl20260630_18B/SigIn/CAN1/DbugBMS_SOC_CaleSOC/UNPACK ==
  ID : Inport
  data : Inport  Port=2
  length : Inport  Port=3
  timestamp : Inport  Port=4
  Action Port : ActionPort  ActionType=case
  Add : Sum
  Bus Creator : BusCreator  Inputs=7  OutDataTypeStr=Bus: CAN_MESSAGE_BUS  NonVirtualBus=on
  Bus Creator1 : BusCreator  Inputs=1
  CAN Unpack6 : canmsglib/CAN Unpack  CANdbFile=D:\VCU\VCU_AgriculturalMachinery_ChangChun\CAN协议8.4\BMS\BMS_DBC_Sheet1.dbc  MsgList=DbugBMS_SOC_CaleSOC  MsgName=DbugBMS_SOC_CaleSOC  MsgIDType=Extended (29-bit identifier)  MsgIdentifier=469857607  MsgLength=8  SignalInfo=APPSOC$12$12$2$2$1$0$1.000000e-01$0$0$100$#  NSignals=1  IDPort=off  TimestampPort=off  ErrorPort=off  RemotePort=off  LengthPort=off  StatusPort=off  StartBits=str2num('[int32(12)]')  SignalSizes=str2num('[int32(12)]')  ByteOrders=str2num('[int32(2)]')  DataTypes=str2num('[int32(2)]')  MultiplexTypes=str2num('[int32(1)]')  MultiplexValues=str2num('[double(0)]')  Factors=str2num('[double(1.000000e-01)]')  Offsets=str2num('[double(0)]')  Minimums=str2num('[double(0)]')  Maximums=str2num('[double(100)]')  ApplyMinMax=off
      settings: SourceProductName=Simulink Real-Time  SourceProductBaseCode=XP  DataFormat=CANdb specified signals
  Constant : Constant  OutDataTypeStr=uint8
  Constant1 : Constant  OutDataTypeStr=uint8
  Constant4 : Constant  Value=0  OutDataTypeStr=uint8
  Constant5 : Constant  Value=0  OutDataTypeStr=uint8
  Data Store Read : DataStoreRead  DataStoreName=Cnt_BMS5
  Data Store Write : DataStoreWrite  DataStoreName=Cnt_BMS5
  Data Type Conversion{,14..15,17} (4 alike) : DataTypeConversion  OutDataTypeStr=uint8
  Data Type Conversion18 : DataTypeConversion  OutDataTypeStr=uint32
  Data Type Conversion19 : DataTypeConversion  OutDataTypeStr=double
  Data Type Conversion60 : DataTypeConversion  OutDataTypeStr=single
  Message : Outport
  wires:
  Constant4/1 -> Data Type Conversion15/1
  length/1 -> Data Type Conversion14/1
  data/1 -> Bus Creator/7  "Data"
  Data Type Conversion18/1 -> Bus Creator/5  "ID"
  Constant1/1 -> Data Type Conversion/1
  Constant5/1 -> Data Type Conversion17/1
  ID/1 -> Data Type Conversion18/1
  Data Type Conversion19/1 -> Bus Creator/6  "Timestamp"
  timestamp/1 -> Data Type Conversion19/1
  Data Type Conversion17/1 -> Bus Creator/4  "Error"
  Bus Creator/1 -> CAN Unpack6/1  "CAN_Msg_In"
  Data Type Conversion/1 -> Bus Creator/1  "Extended"
  Data Type Conversion14/1 -> Bus Creator/2  "Length"
  Data Type Conversion15/1 -> Bus Creator/3  "Remote"
  Bus Creator1/1 -> Message/1
  Data Type Conversion60/1 -> Bus Creator1/1  "APPSOC"
  CAN Unpack6/1 -> Data Type Conversion60/1
  Add/1 -> Data Store Write/1
  Constant/1 -> Add/2
  Data Store Read/1 -> Add/1

== system VehCtrl20260630_18B/SigIn/CAN1/MCU2VCU_1/UNPACK ==
  ID : Inport
  data : Inport  Port=2
  length : Inport  Port=3
  timestamp : Inport  Port=4
  Action Port : ActionPort  ActionType=case
  Add : Sum
  Bus Creator : BusCreator  Inputs=7  OutDataTypeStr=Bus: CAN_MESSAGE_BUS  NonVirtualBus=on
  Bus Creator1 : BusCreator  Inputs=14
  CAN Unpack6 : canmsglib/CAN Unpack  CANdbFile=D:\VCU\VCU_AgriculturalMachinery_ChangChun\CAN协议8.4\MCU\MCU_Sheet1.dbc  MsgList=MCU_VCU_FL_1  MsgName=MCU_VCU_FL_1  MsgIDType=Extended (29-bit identifier)  MsgIdentifier=201893875  MsgLength=8  SignalInfo=MCU_Canlife$60$4$1$2$1$0$1$0$0$15$#MCU_ContactorStatus$56$2$1$2$1$0$1$0$0$3$#MCU_Gear$58$2$1$2$1$0$1$0$0$3$#MCU_SpdEst$16$16$1$2$1$0$1$-32000$-32000$33535$#MCU_TrqEst$0$16$1$2$1$0$1.000000e-01$-3200$-3200$3.353500e+03$#MCU_WorkStatus$48$8$1$2$1$0$1$0$0$255$#MCU_nCurrent$32$16$1$2$1$0$1.000000e-01$-3200$-3200$3.353500e+03$#  NSignals=7  IDPort=off  TimestampPort=off  ErrorPort=off  RemotePort=off  LengthPort=off  StatusPort=off  StartBits=str2num('[int32(60);int32(56);int32(58);int32(16);int32(0);int32(48);int32(32)]')  SignalSizes=str2num('[int32(4);int32(2);int32(2);int32(16);int32(16);int32(8);int32(16)]')  ByteOrders=str2num('[int32(1);int32(1);int32(1);int32(1);int32(1);int32(1);int32(1)]')  DataTypes=str2num('[int32(2);int32(2);int32(2);int32(2);int32(2);int32(2);int32(2)]')  MultiplexTypes=str2num('[int32(1);int32(1);int32(1);int32(1);int32(1);int32(1);int32(1)]')  MultiplexValues=str2num('[double(0);double(0);double(0);double(0);double(0);double(0);double(0)]')  Factors=str2num('[double(1);double(1);double(1);double(1);double(1.000000e-01);double(1);double(1.000000e-01)]')  Offsets=str2num('[double(0);double(0);double(0);double(-32000);double(-3200);double(0);double(-3200)]')  Minimums=str2num('[double(0);double(0);double(0);double(-32000);double(-3200);double(0);double(-3200)]')  Maximums=str2num('[double(15);double(3);double(3);double(33535);double(3.353500e+03);double(255);double(3.353500e+03)]')  ApplyMinMax=off
      settings: SourceProductName=Simulink Real-Time  SourceProductBaseCode=XP  DataFormat=CANdb specified signals
  Constant : Constant  OutDataTypeStr=uint8
  Constant1 : Constant  OutDataTypeStr=uint8
  Constant4 : Constant  Value=0  OutDataTypeStr=uint8
  Constant5 : Constant  Value=0  OutDataTypeStr=uint8
  Data Store Read : DataStoreRead  DataStoreName=Cnt_MCU1_1
  Data Store Write : DataStoreWrite  DataStoreName=Cnt_MCU1_1
  Data Store Write1 : DataStoreWrite  DataStoreName=MtrSpdFL
  Data Type Conversion{,1..4,14..15,17} (8 alike) : DataTypeConversion  OutDataTypeStr=uint8
  Data Type Conversion18 : DataTypeConversion  OutDataTypeStr=uint32
  Data Type Conversion19 : DataTypeConversion  OutDataTypeStr=double
  Data Type Conversion60 : DataTypeConversion  OutDataTypeStr=single
  Data Type Conversion61 : DataTypeConversion  OutDataTypeStr=single
  Data Type Conversion62 : DataTypeConversion  OutDataTypeStr=single
  Gain : Gain  Gain=-1
  Subsystem : Subsystem
  Message : Outport
  wires:
  Constant4/1 -> Data Type Conversion15/1
  length/1 -> Data Type Conversion14/1
  data/1 -> Bus Creator/7  "Data"
  Data Type Conversion18/1 -> Bus Creator/5  "ID"
  Constant1/1 -> Data Type Conversion/1
  Constant5/1 -> Data Type Conversion17/1
  ID/1 -> Data Type Conversion18/1
  Data Type Conversion19/1 -> Bus Creator/6  "Timestamp"
  timestamp/1 -> Data Type Conversion19/1
  Data Type Conversion17/1 -> Bus Creator/4  "Error"
  Bus Creator/1 -> CAN Unpack6/1  "CAN_Msg_In"
  Data Type Conversion/1 -> Bus Creator/1  "Extended"
  Data Type Conversion14/1 -> Bus Creator/2  "Length"
  Data Type Conversion15/1 -> Bus Creator/3  "Remote"
  Bus Creator1/1 -> Message/1
  Data Type Conversion60/1 -> Bus Creator1/5  "MCU_TrqEst"
  Data Type Conversion61/1 -> Gain/1
  Data Type Conversion62/1 -> Bus Creator1/6  "MCU_nCurrent"
  Data Type Conversion1/1 -> Bus Creator1/1  "MCU_Canlife"
  CAN Unpack6/6 -> Data Type Conversion2/1
  CAN Unpack6/1 -> Data Type Conversion1/1
  CAN Unpack6/5 -> Data Type Conversion60/1
  CAN Unpack6/4 -> Data Type Conversion61/1
  CAN Unpack6/7 -> Data Type Conversion62/1
  CAN Unpack6/2 -> Data Type Conversion3/1
  CAN Unpack6/3 -> Data Type Conversion4/1
  Data Type Conversion3/1 -> Bus Creator1/2  "MCU_ContactorStatus"
  Data Type Conversion4/1 -> Bus Creator1/3  "MCU_Gear"
  Gain/1 -> Data Store Write1/1, Bus Creator1/4  "MCU_SpdEst"
  Data Type Conversion2/1 -> Subsystem/1(WorkStatus)  "MCU_WorkStatus"
  Subsystem/1(StartORStop) -> Bus Creator1/7  "MCU_StartORStop"
  Subsystem/2(Discharge) -> Bus Creator1/8  "MCU_Discharge"
  Subsystem/3(Direction) -> Bus Creator1/9  "MCU_Direction"
  Subsystem/4(DrvORBrk) -> Bus Creator1/10  "MCU_DrvORBrk"
  Subsystem/5(Fault) -> Bus Creator1/11  "MCU_Fault"
  Subsystem/6(Ready) -> Bus Creator1/12  "MCU_Ready"
  Subsystem/7(Mode) -> Bus Creator1/13  "MCU_Mode"
  Subsystem/8(PWM) -> Bus Creator1/14  "MCU_PWM"
  Data Store Read/1 -> Add/1
  Constant/1 -> Add/2
  Add/1 -> Data Store Write/1

== system VehCtrl20260630_18B/SigIn/CAN1/MCU2VCU_10/UNPACK ==
  ID : Inport
  data : Inport  Port=2
  length : Inport  Port=3
  timestamp : Inport  Port=4
  Action Port : ActionPort  ActionType=case
  Add : Sum
  Bus Creator : BusCreator  Inputs=7  OutDataTypeStr=Bus: CAN_MESSAGE_BUS  NonVirtualBus=on
  Bus Creator1 : BusCreator  Inputs=5
  CAN Unpack6 : canmsglib/CAN Unpack  CANdbFile=D:\VCU\VCU_AgriculturalMachinery_ChangChun\CAN协议8.4\MCU\MCU_Sheet1.dbc  MsgList=MCU_VCU_FR_2  MsgName=MCU_VCU_FR_2  MsgIDType=Extended (29-bit identifier)  MsgIdentifier=201959408  MsgLength=8  SignalInfo=MCU_AC_Voltage$16$16$1$2$1$0$1.000000e-01$0$0$6.553500e+03$#MCU_DC_Voltage$0$16$1$2$1$0$1.000000e-01$0$0$6.553500e+03$#MCU_nAvailI$32$16$1$2$1$0$1.000000e-01$0$0$6.553500e+03$#MCU_nControllerTemp$48$8$1$2$1$0$1$-40$-40$215$#MCU_nMotorTemp$56$8$1$2$1$0$1$-40$-40$215$#  NSignals=5  IDPort=off  TimestampPort=off  ErrorPort=off  RemotePort=off  LengthPort=off  StatusPort=off  StartBits=str2num('[int32(16);int32(0);int32(32);int32(48);int32(56)]')  SignalSizes=str2num('[int32(16);int32(16);int32(16);int32(8);int32(8)]')  ByteOrders=str2num('[int32(1);int32(1);int32(1);int32(1);int32(1)]')  DataTypes=str2num('[int32(2);int32(2);int32(2);int32(2);int32(2)]')  MultiplexTypes=str2num('[int32(1);int32(1);int32(1);int32(1);int32(1)]')  MultiplexValues=str2num('[double(0);double(0);double(0);double(0);double(0)]')  Factors=str2num('[double(1.000000e-01);double(1.000000e-01);double(1.000000e-01);double(1);double(1)]')  Offsets=str2num('[double(0);double(0);double(0);double(-40);double(-40)]')  Minimums=str2num('[double(0);double(0);double(0);double(-40);double(-40)]')  Maximums=str2num('[double(6.553500e+03);double(6.553500e+03);double(6.553500e+03);double(215);double(215)]')  ApplyMinMax=off
      settings: SourceProductName=Simulink Real-Time  SourceProductBaseCode=XP  DataFormat=CANdb specified signals
  Constant : Constant  OutDataTypeStr=uint8
  Constant1 : Constant  OutDataTypeStr=uint8
  Constant4 : Constant  Value=0  OutDataTypeStr=uint8
  Constant5 : Constant  Value=0  OutDataTypeStr=uint8
  Data Store Read : DataStoreRead  DataStoreName=Cnt_MCU2_2
  Data Store Write : DataStoreWrite  DataStoreName=Cnt_MCU2_2
  Data Store Write2 : DataStoreWrite  DataStoreName=MtrMotorTempFR
  Data Store Write3 : DataStoreWrite  DataStoreName=MtrControlerTempFR
  Data Type Conversion{,14..15,17} (4 alike) : DataTypeConversion  OutDataTypeStr=uint8
  Data Type Conversion{1,60..63} (5 alike) : DataTypeConversion  OutDataTypeStr=single
  Data Type Conversion18 : DataTypeConversion  OutDataTypeStr=uint32
  Data Type Conversion19 : DataTypeConversion  OutDataTypeStr=double
  Message : Outport
  wires:
  Constant4/1 -> Data Type Conversion15/1
  length/1 -> Data Type Conversion14/1
  data/1 -> Bus Creator/7  "Data"
  Data Type Conversion18/1 -> Bus Creator/5  "ID"
  Constant1/1 -> Data Type Conversion/1
  Constant5/1 -> Data Type Conversion17/1
  ID/1 -> Data Type Conversion18/1
  Data Type Conversion19/1 -> Bus Creator/6  "Timestamp"
  timestamp/1 -> Data Type Conversion19/1
  Data Type Conversion17/1 -> Bus Creator/4  "Error"
  Bus Creator/1 -> CAN Unpack6/1  "CAN_Msg_In"
  Data Type Conversion/1 -> Bus Creator/1  "Extended"
  Data Type Conversion14/1 -> Bus Creator/2  "Length"
  Data Type Conversion15/1 -> Bus Creator/3  "Remote"
  Bus Creator1/1 -> Message/1
  Data Type Conversion60/1 -> Bus Creator1/1  "MCU_DC_Voltage"
  Data Type Conversion61/1 -> Bus Creator1/2  "MCU_AC_Voltage"
  Data Type Conversion62/1 -> Bus Creator1/3  "MCU_nAvailI"
  Data Type Conversion63/1 -> Data Store Write3/1, Bus Creator1/4  "MCU_nControllerTemp"
  Data Type Conversion1/1 -> Data Store Write2/1, Bus Creator1/5  "MCU_nMotorTemp"
  CAN Unpack6/1 -> Data Type Conversion61/1  "MCU_FaultLevel"
  CAN Unpack6/2 -> Data Type Conversion60/1  "MCU_FaultNumber"
  CAN Unpack6/3 -> Data Type Conversion62/1
  CAN Unpack6/4 -> Data Type Conversion63/1
  CAN Unpack6/5 -> Data Type Conversion1/1
  Data Store Read/1 -> Add/1
  Add/1 -> Data Store Write/1
  Constant/1 -> Add/2
